simulink model "lews_model"  (R2026a)
settings: Solver=ode45  StopTime=Inf
libraries: simulink x4
settings Model: Creator=HARIKRISHNAN  LastModifiedBy=HARIKRISHNAN

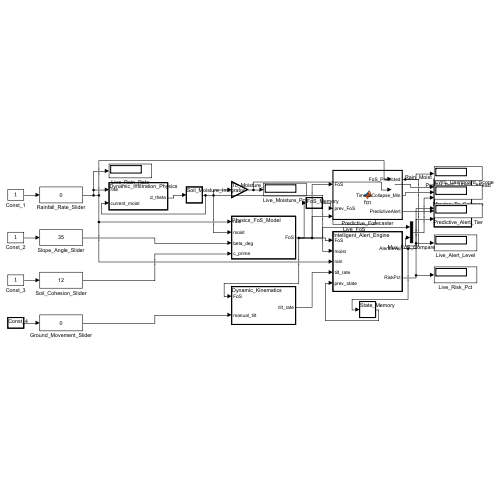
[thumbnail: Simulink's stored preview of the top-level diagram]
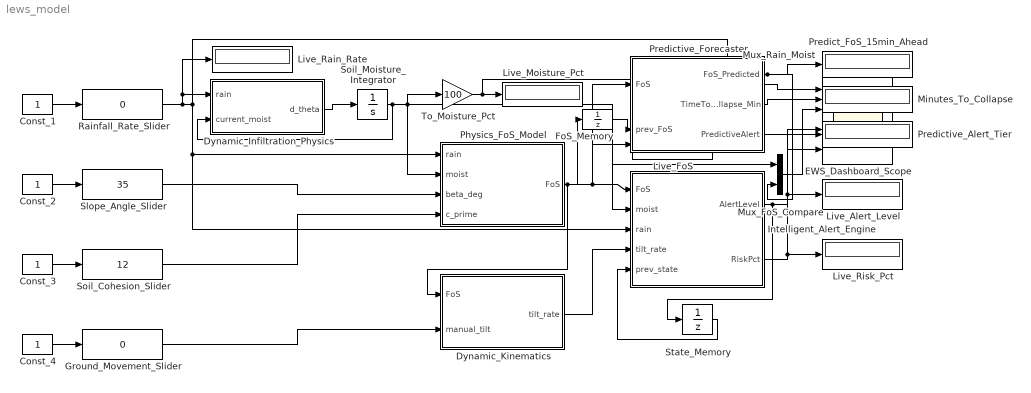
== system lews_model ==
  Const_{1..4} (4 alike) : Constant
  Dynamic_Infiltration_Physics : MATLAB Function  TreatAsAtomicUnit=on
  Dynamic_Kinematics : MATLAB Function  TreatAsAtomicUnit=on
  EWS_Dashboard_Scope : Scope  NumInputPorts=4
      settings: Title=2. PREDICTIVE FORECAST: Current FoS (Yellow) vs 15-Min Predicted FoS (Magenta)  ActiveDisplayYMinimum=0  ActiveDisplayYMaximum=2.5
  FoS_Memory : UnitDelay  InitialCondition=1.8  SampleTime=0.5
  Ground_Movement_Slider : simulink/Math Operations/Slider Gain  gain=0  low=0  high=10
  Intelligent_Alert_Engine : MATLAB Function  TreatAsAtomicUnit=on
  Live_Alert_Level : Display
  Live_FoS : Display
  Live_Moisture_Pct : Display
  Live_Rain_Rate : Display
  Live_Risk_Pct : Display
  Minutes_To_Collapse : Display
  Mux_FoS_Compare : Mux  Inputs=2
  Mux_Rain_Moist : Mux  Inputs=2
  Physics_FoS_Model : MATLAB Function  TreatAsAtomicUnit=on
  Predict_FoS_15min_Ahead : Display
  Predictive_Alert_Tier : Display
  Predictive_Forecaster : MATLAB Function  TreatAsAtomicUnit=on
  Rainfall_Rate_Slider : simulink/Math Operations/Slider Gain  gain=0  low=0  high=100
  Slope_Angle_Slider : simulink/Math Operations/Slider Gain  gain=35  low=20  high=50
  Soil_Cohesion_Slider : simulink/Math Operations/Slider Gain  gain=12  low=5  high=30
  Soil_Moisture_Integrator : Integrator  InitialCondition=0.18  LimitOutput=on  UpperSaturationLimit=0.58  LowerSaturationLimit=0.15
  State_Memory : UnitDelay  SampleTime=0.1
  To_Moisture_Pct : Gain  Gain=100
  wires:
  Const_1/1 -> Rainfall_Rate_Slider/1
  Const_2/1 -> Slope_Angle_Slider/1
  Const_3/1 -> Soil_Cohesion_Slider/1
  Const_4/1 -> Ground_Movement_Slider/1
  Rainfall_Rate_Slider/1 -> Physics_FoS_Model/1(rain), Intelligent_Alert_Engine/3(rain), Mux_Rain_Moist/1, Dynamic_Infiltration_Physics/1(rain), Live_Rain_Rate/1
  Dynamic_Infiltration_Physics/1(d_theta) -> Soil_Moisture_Integrator/1
  Soil_Moisture_Integrator/1 -> Physics_FoS_Model/2(moist), Intelligent_Alert_Engine/2(moist), To_Moisture_Pct/1, Dynamic_Infiltration_Physics/2(current_moist)
  Slope_Angle_Slider/1 -> Physics_FoS_Model/3(beta_deg)
  Soil_Cohesion_Slider/1 -> Physics_FoS_Model/4(c_prime)
  Physics_FoS_Model/1(FoS) -> Live_FoS/1, Intelligent_Alert_Engine/1(FoS), Dynamic_Kinematics/1(FoS), Predictive_Forecaster/1(FoS), FoS_Memory/1, Mux_FoS_Compare/1
  Ground_Movement_Slider/1 -> Dynamic_Kinematics/2(manual_tilt)
  Dynamic_Kinematics/1(tilt_rate) -> Intelligent_Alert_Engine/4(tilt_rate)
  To_Moisture_Pct/1 -> Live_Moisture_Pct/1, Mux_Rain_Moist/2
  Intelligent_Alert_Engine/2(RiskPct) -> Live_Risk_Pct/1, EWS_Dashboard_Scope/3
  Intelligent_Alert_Engine/1(AlertLevel) -> Live_Alert_Level/1, EWS_Dashboard_Scope/4, State_Memory/1
  Mux_Rain_Moist/1 -> EWS_Dashboard_Scope/1
  State_Memory/1 -> Intelligent_Alert_Engine/5(prev_state)
  FoS_Memory/1 -> Predictive_Forecaster/2(prev_FoS)
  Predictive_Forecaster/1(FoS_Predicted) -> Predict_FoS_15min_Ahead/1, Mux_FoS_Compare/2
  Predictive_Forecaster/2(TimeToCollapse_Min) -> Minutes_To_Collapse/1
  Predictive_Forecaster/3(PredictiveAlert) -> Predictive_Alert_Tier/1
  Mux_FoS_Compare/1 -> EWS_Dashboard_Scope/2

== matlab function lews_model/Physics_FoS_Model ==
  data: rain input; FoS output; moist input; beta_deg input; c_prime input
function FoS = Physics_FoS_Model(rain, moist, beta_deg, c_prime)
% Geotechnical Constants
phi_rad = deg2rad(30);
beta_rad = deg2rad(beta_deg);
gamma_s = 18;     % kN/m^3
gamma_w = 9.81;   % kN/m^3
z = 1.5;          % meters

% Dynamic Pore-water pressure (u in kPa)
theta_crit = 0.35;
if moist > theta_crit
    u = gamma_w * (moist - theta_crit) * z * 3.0 + (rain * 0.02);
else
    u = 0;
end

normal_stress = gamma_s * z * (cos(beta_rad))^2;
eff_stress = max(normal_stress - u, 0.05);
resisting_shear = c_prime + eff_stress * tan(phi_rad);
driving_shear = gamma_s * z * sin(beta_rad) * cos(beta_rad);
FoS = resisting_shear / max(driving_shear, 0.001);
end

== matlab function lews_model/Dynamic_Infiltration_Physics ==
  data: rain input; d_theta output; current_moist input
function d_theta = Dynamic_Infiltration_Physics(rain, current_moist)
r = double(rain);
cm = double(current_moist);
infil = (r / 100) * 0.008;
drainage = 0.001 * max(0, cm - 0.18);
d_theta = double(infil - drainage);
end

== matlab function lews_model/Dynamic_Kinematics ==
  data: FoS input; tilt_rate output; manual_tilt input
function tilt_rate = Dynamic_Kinematics(FoS, manual_tilt)
f = double(FoS);
mt = double(manual_tilt);
if f > 1.30
    auto_creep = 0.05;
elseif f > 1.05
    auto_creep = (1.30 - f) * 6.0;
else
    auto_creep = 1.5 + (1.05 - f) * 20.0;
end
tilt_rate = double(auto_creep + mt);
end

== matlab function lews_model/Intelligent_Alert_Engine ==
  data: FoS input; AlertLevel output; moist input; rain input; tilt_rate input; RiskPct output; prev_state input
function [AlertLevel, RiskPct] = Intelligent_Alert_Engine(FoS, moist, rain, tilt_rate, prev_state)
f = double(FoS);
m = double(moist);
r = double(rain);
tr = double(tilt_rate);
ps = double(prev_state);

% Continuous Risk % (0 to 100%)
fos_risk = max(0, min(100, (1.6 - f) * 120));
kinematic_risk = min(100, tr * 25);
moist_risk = max(0, (m - 0.25) * 280);
RiskPct = max(0, min(100, 0.45*fos_risk + 0.35*kinematic_risk + 0.20*moist_risk));

% Multi-tier Warning Levels with Hysteresis
current_state = ps;
if ps == 0
    if RiskPct >= 45 || f < 1.15 || tr > 3.0
        current_state = 1;
    end
elseif ps == 1
    if RiskPct >= 75 || f < 1.0 || (f < 1.1 && tr > 2.5)
        current_state = 2;
    elseif RiskPct < 30 && f > 1.30 && tr < 1.0
        current_state = 0;
    end
elseif ps == 2
    if RiskPct < 55 && f > 1.25
        current_state = 1;
    end
end
AlertLevel = double(current_state);
end

== matlab function lews_model/Predictive_Forecaster ==
  data: FoS input; FoS_Predicted output; prev_FoS input; TimeToCollapse_Min output; PredictiveAlert output
function [FoS_Predicted, TimeToCollapse_Min, PredictiveAlert] = Predictive_Forecaster(FoS, prev_FoS)
% Forecasts slope failure 15 to 30 minutes before catastrophic collapse
f = double(FoS);
pf = double(prev_FoS);

% Calculate stability trend rate (change per second)
% Sample time of feedback is dt = 0.5s
dt = 0.5;
rate_of_change = (f - pf) / dt; % d(FoS)/dt

% Extrapolate 15 minutes (900 seconds) into the future
lead_time_sec = 900;
FoS_Predicted = max(0, min(3.0, f + (rate_of_change * lead_time_sec)));

% Calculate Estimated Time-to-Failure (TTF in minutes)
% Failure occurs when FoS reaches 1.0
if rate_of_change < -0.00005 && f > 1.0
    ttf_sec = (f - 1.0) / (-rate_of_change);
    TimeToCollapse_Min = max(0, min(120, ttf_sec / 60));
elseif f <= 1.0
    TimeToCollapse_Min = 0; % Already failing
else
    TimeToCollapse_Min = 999; % Slope is stable or recovering
end

% Predictive Early Warning Level
% 0 = Safe, 1 = Predicted Collapse in < 30 min, 2 = Imminent Failure in < 10 min
if TimeToCollapse_Min < 10 || f < 1.0
    PredictiveAlert = 2; % EVACUATE
elseif TimeToCollapse_Min < 35 || FoS_Predicted < 1.05
    PredictiveAlert = 1; % PREDICTIVE ADVISORY (ADVANCE WARNING)
else
    PredictiveAlert = 0; % SAFE
end
end
